simulink model "sh1"  (Simulink 6.6)
settings: Solver=ode45  StartTime=0.0  StopTime=10.0  RelTol=1e-3
libraries: cdsFilt x66, cdsEpicsIn x10, cdsWD x7, cdsMuxMatrix x4, cdsEpicsOut x2, cdsDio x2, dac x1, cdsEpicsBinIn x1, cdsParameters x1
(part 4 of 4)

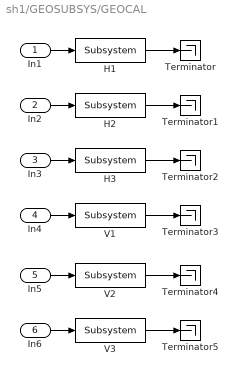
== system sh1/GEOSUBSYS/GEOCAL ==
  In1 : Inport
  In2 : Inport  Port=2
  In3 : Inport  Port=3
  In4 : Inport  Port=4
  In5 : Inport  Port=5
  In6 : Inport  Port=6
  H1 : cdsFilt/Subsystem  Tag=cdsFilt  Description=|  SystemSampleTime=-1
      | Purpose:                                                                                                                                                                                                                                  
      | Standard CDS IIR filter module.                                                                                                                                                                                                           
      |                                                                                                                                                                                                                                           
      | Operation:                                                                                                                                                                                                                                
      | Consists of 10 second order section IIR filters, plus a ramped gain stage. In FE code, also provides pre-defined test points and excitation channel inputs. The filter coefficients are defined in the LIGO system using the 'foton' tool.
      |                                                                                                                                                                                                                                           
      | Usage:                                                                                                                                                                                                                                    
      | Name the part with the desired filter module name.
      settings: AttributesFormatString=%<Tag>
  H2 : cdsFilt/Subsystem  Tag=cdsFilt  Description=|  SystemSampleTime=-1
      | Purpose:                                                                                                                                                                                                                                  
      | Standard CDS IIR filter module.                                                                                                                                                                                                           
      |                                                                                                                                                                                                                                           
      | Operation:                                                                                                                                                                                                                                
      | Consists of 10 second order section IIR filters, plus a ramped gain stage. In FE code, also provides pre-defined test points and excitation channel inputs. The filter coefficients are defined in the LIGO system using the 'foton' tool.
      |                                                                                                                                                                                                                                           
      | Usage:                                                                                                                                                                                                                                    
      | Name the part with the desired filter module name.
      settings: AttributesFormatString=%<Tag>
  H3 : cdsFilt/Subsystem  Tag=cdsFilt  Description=|  SystemSampleTime=-1
      | Purpose:                                                                                                                                                                                                                                  
      | Standard CDS IIR filter module.                                                                                                                                                                                                           
      |                                                                                                                                                                                                                                           
      | Operation:                                                                                                                                                                                                                                
      | Consists of 10 second order section IIR filters, plus a ramped gain stage. In FE code, also provides pre-defined test points and excitation channel inputs. The filter coefficients are defined in the LIGO system using the 'foton' tool.
      |                                                                                                                                                                                                                                           
      | Usage:                                                                                                                                                                                                                                    
      | Name the part with the desired filter module name.
      settings: AttributesFormatString=%<Tag>
  Terminator{,1..5} (6 alike) : Terminator
  V1 : cdsFilt/Subsystem  Tag=cdsFilt  Description=|  SystemSampleTime=-1
      | Purpose:                                                                                                                                                                                                                                  
      | Standard CDS IIR filter module.                                                                                                                                                                                                           
      |                                                                                                                                                                                                                                           
      | Operation:                                                                                                                                                                                                                                
      | Consists of 10 second order section IIR filters, plus a ramped gain stage. In FE code, also provides pre-defined test points and excitation channel inputs. The filter coefficients are defined in the LIGO system using the 'foton' tool.
      |                                                                                                                                                                                                                                           
      | Usage:                                                                                                                                                                                                                                    
      | Name the part with the desired filter module name.
      settings: AttributesFormatString=%<Tag>
  V2 : cdsFilt/Subsystem  Tag=cdsFilt  Description=|  SystemSampleTime=-1
      | Purpose:                                                                                                                                                                                                                                  
      | Standard CDS IIR filter module.                                                                                                                                                                                                           
      |                                                                                                                                                                                                                                           
      | Operation:                                                                                                                                                                                                                                
      | Consists of 10 second order section IIR filters, plus a ramped gain stage. In FE code, also provides pre-defined test points and excitation channel inputs. The filter coefficients are defined in the LIGO system using the 'foton' tool.
      |                                                                                                                                                                                                                                           
      | Usage:                                                                                                                                                                                                                                    
      | Name the part with the desired filter module name.
      settings: AttributesFormatString=%<Tag>
  V3 : cdsFilt/Subsystem  Tag=cdsFilt  Description=|  SystemSampleTime=-1
      | Purpose:                                                                                                                                                                                                                                  
      | Standard CDS IIR filter module.                                                                                                                                                                                                           
      |                                                                                                                                                                                                                                           
      | Operation:                                                                                                                                                                                                                                
      | Consists of 10 second order section IIR filters, plus a ramped gain stage. In FE code, also provides pre-defined test points and excitation channel inputs. The filter coefficients are defined in the LIGO system using the 'foton' tool.
      |                                                                                                                                                                                                                                           
      | Usage:                                                                                                                                                                                                                                    
      | Name the part with the desired filter module name.
      settings: AttributesFormatString=%<Tag>
  wires:
  V2/1 -> Terminator4/1
  V3/1 -> Terminator5/1
  In6/1 -> V3/1
  In5/1 -> V2/1
  H3/1 -> Terminator2/1
  V1/1 -> Terminator3/1
  In4/1 -> V1/1
  In3/1 -> H3/1
  H1/1 -> Terminator/1
  H2/1 -> Terminator1/1
  In2/1 -> H2/1
  In1/1 -> H1/1

== system sh1/WD/1 ==
  In1 : Inport
  In2 : Inport  Port=2
  In3 : Inport  Port=3
  In4 : Inport  Port=4
  In5 : Inport  Port=5
  In6 : Inport  Port=6
  Gain : Gain  Gain=1000
  Ground : Ground
  MAX : cdsEpicsIn/Subsystem  Tag=cdsEpicsIn  Description=|  SystemSampleTime=-1
      | Purpose:                                                                              
      | Create an EPICS input channel connection to the FE realtime controls.                 
      |                                                                                       
      | Operation:                                                                            
      | Outputs value from an EPICS ai record. Value is floating point with a precision of 3..
      |                                                                                       
      | Usage:                                                                                
      | Name the part with the desired EPICS channel name.
      settings: AttributesFormatString=%<Tag>
  Operator{1,3..6} (5 alike) : RelationalOperator  Operator=>  LogicOutDataTypeMode=Boolean
  Operator2 : RelationalOperator  Operator=>  LogicOutDataTypeMode=Boolean  ZeroCross=off
  SWITCH : cdsWD/Subsystem  Description=cdsWD  SystemSampleTime=-1
      settings: AttributesFormatString=%<Description>
  Sum1 : Sum  Inputs=6
  Out1 : Outport
  wires:
  In1/1 -> Operator1/1
  In2/1 -> Operator2/1
  In3/1 -> Operator3/1
  In4/1 -> Operator4/1
  In5/1 -> Operator5/1
  In6/1 -> Operator6/1
  Operator1/1 -> Sum1/1
  Operator2/1 -> Sum1/2
  Operator3/1 -> Sum1/3
  Operator4/1 -> Sum1/4
  Operator5/1 -> Sum1/5
  Operator6/1 -> Sum1/6
  MAX/1 -> Operator1/2, Operator2/2, Operator3/2, Operator4/2, Operator5/2, Operator6/2
  SWITCH/1 -> Out1/1
  Sum1/1 -> Gain/1
  Ground/1 -> SWITCH/2, SWITCH/3, SWITCH/5, SWITCH/4
  Gain/1 -> SWITCH/1

== system sh1/WD/2 ==
  In1 : Inport
  In2 : Inport  Port=2
  In3 : Inport  Port=3
  In4 : Inport  Port=4
  In5 : Inport  Port=5
  In6 : Inport  Port=6
  Gain : Gain  Gain=1000
  Ground : Ground
  MAX : cdsEpicsIn/Subsystem  Tag=cdsEpicsIn  Description=|  SystemSampleTime=-1
      | Purpose:                                                                              
      | Create an EPICS input channel connection to the FE realtime controls.                 
      |                                                                                       
      | Operation:                                                                            
      | Outputs value from an EPICS ai record. Value is floating point with a precision of 3..
      |                                                                                       
      | Usage:                                                                                
      | Name the part with the desired EPICS channel name.
      settings: AttributesFormatString=%<Tag>
  Operator{1..6} (6 alike) : RelationalOperator  Operator=>  LogicOutDataTypeMode=Boolean
  SWITCH : cdsWD/Subsystem  Description=cdsWD  SystemSampleTime=-1
      settings: AttributesFormatString=%<Description>
  Sum1 : Sum  Inputs=6
  Out1 : Outport
  wires:
  In1/1 -> Operator1/1
  In2/1 -> Operator2/1
  In3/1 -> Operator3/1
  In4/1 -> Operator4/1
  In5/1 -> Operator5/1
  In6/1 -> Operator6/1
  Operator1/1 -> Sum1/1
  Operator2/1 -> Sum1/2
  Operator3/1 -> Sum1/3
  Operator4/1 -> Sum1/4
  Operator5/1 -> Sum1/5
  Operator6/1 -> Sum1/6
  MAX/1 -> Operator1/2, Operator2/2, Operator3/2, Operator4/2, Operator5/2, Operator6/2
  SWITCH/1 -> Out1/1
  Ground/1 -> SWITCH/2, SWITCH/3, SWITCH/5, SWITCH/4
  Sum1/1 -> Gain/1
  Gain/1 -> SWITCH/1

== system sh1/WD/3 ==
  In1 : Inport
  In2 : Inport  Port=2
  In3 : Inport  Port=3
  In4 : Inport  Port=4
  In5 : Inport  Port=5
  In6 : Inport  Port=6
  Gain : Gain  Gain=1000
  Ground : Ground
  MAX : cdsEpicsIn/Subsystem  Tag=cdsEpicsIn  Description=|  SystemSampleTime=-1
      | Purpose:                                                                              
      | Create an EPICS input channel connection to the FE realtime controls.                 
      |                                                                                       
      | Operation:                                                                            
      | Outputs value from an EPICS ai record. Value is floating point with a precision of 3..
      |                                                                                       
      | Usage:                                                                                
      | Name the part with the desired EPICS channel name.
      settings: AttributesFormatString=%<Tag>
  Operator{1..6} (6 alike) : RelationalOperator  Operator=>  LogicOutDataTypeMode=Boolean
  SWITCH : cdsWD/Subsystem  Description=cdsWD  SystemSampleTime=-1
      settings: AttributesFormatString=%<Description>
  Sum1 : Sum  Inputs=6
  Out1 : Outport
  wires:
  In1/1 -> Operator1/1
  In2/1 -> Operator2/1
  In3/1 -> Operator3/1
  In4/1 -> Operator4/1
  In5/1 -> Operator5/1
  In6/1 -> Operator6/1
  Operator1/1 -> Sum1/1
  Operator2/1 -> Sum1/2
  Operator3/1 -> Sum1/3
  Operator4/1 -> Sum1/4
  Operator5/1 -> Sum1/5
  Operator6/1 -> Sum1/6
  MAX/1 -> Operator1/2, Operator2/2, Operator3/2, Operator4/2, Operator5/2, Operator6/2
  SWITCH/1 -> Out1/1
  Ground/1 -> SWITCH/2, SWITCH/3, SWITCH/5, SWITCH/4
  Sum1/1 -> Gain/1
  Gain/1 -> SWITCH/1

== system sh1/WD/4 ==
  In1 : Inport
  In2 : Inport  Port=2
  In3 : Inport  Port=3
  Gain : Gain  Gain=1000
  Ground : Ground
  MAX : cdsEpicsIn/Subsystem  Tag=cdsEpicsIn  Description=|  SystemSampleTime=-1
      | Purpose:                                                                              
      | Create an EPICS input channel connection to the FE realtime controls.                 
      |                                                                                       
      | Operation:                                                                            
      | Outputs value from an EPICS ai record. Value is floating point with a precision of 3..
      |                                                                                       
      | Usage:                                                                                
      | Name the part with the desired EPICS channel name.
      settings: AttributesFormatString=%<Tag>
  Operator1 : RelationalOperator  Operator=>  LogicOutDataTypeMode=Boolean
  Operator2 : RelationalOperator  Operator=>  LogicOutDataTypeMode=Boolean
  Operator3 : RelationalOperator  Operator=>  LogicOutDataTypeMode=Boolean  ZeroCross=off
  SWITCH : cdsWD/Subsystem  Description=cdsWD  SystemSampleTime=-1
      settings: AttributesFormatString=%<Description>
  Sum1 : Sum  Inputs=3
  Out1 : Outport
  wires:
  In1/1 -> Operator1/1
  In2/1 -> Operator2/1
  In3/1 -> Operator3/1
  Operator1/1 -> Sum1/1
  Operator2/1 -> Sum1/2
  Operator3/1 -> Sum1/3
  MAX/1 -> Operator1/2, Operator2/2, Operator3/2
  SWITCH/1 -> Out1/1
  Ground/1 -> SWITCH/2, SWITCH/3, SWITCH/5, SWITCH/4
  Sum1/1 -> Gain/1
  Gain/1 -> SWITCH/1

== system sh1/WD/5 ==
  In1 : Inport
  In2 : Inport  Port=2
  Gain : Gain  Gain=1000
  Ground : Ground
  MAX : cdsEpicsIn/Subsystem  Tag=cdsEpicsIn  Description=|  SystemSampleTime=-1
      | Purpose:                                                                              
      | Create an EPICS input channel connection to the FE realtime controls.                 
      |                                                                                       
      | Operation:                                                                            
      | Outputs value from an EPICS ai record. Value is floating point with a precision of 3..
      |                                                                                       
      | Usage:                                                                                
      | Name the part with the desired EPICS channel name.
      settings: AttributesFormatString=%<Tag>
  Operator1 : RelationalOperator  Operator=>  LogicOutDataTypeMode=Boolean
  Operator2 : RelationalOperator  Operator=>  LogicOutDataTypeMode=Boolean
  SWITCH : cdsWD/Subsystem  Description=cdsWD  SystemSampleTime=-1
      settings: AttributesFormatString=%<Description>
  Sum1 : Sum  Inputs=2
  Out1 : Outport
  wires:
  In1/1 -> Operator1/1
  In2/1 -> Operator2/1
  Operator1/1 -> Sum1/1
  Operator2/1 -> Sum1/2
  MAX/1 -> Operator1/2, Operator2/2
  SWITCH/1 -> Out1/1
  Ground/1 -> SWITCH/2, SWITCH/3, SWITCH/5, SWITCH/4
  Sum1/1 -> Gain/1
  Gain/1 -> SWITCH/1

== system sh1/WD/6 ==
  In1 : Inport
  In2 : Inport  Port=2
  In3 : Inport  Port=3
  In4 : Inport  Port=4
  Gain : Gain  Gain=1000
  Ground : Ground
  MAX : cdsEpicsIn/Subsystem  Tag=cdsEpicsIn  Description=|  SystemSampleTime=-1
      | Purpose:                                                                              
      | Create an EPICS input channel connection to the FE realtime controls.                 
      |                                                                                       
      | Operation:                                                                            
      | Outputs value from an EPICS ai record. Value is floating point with a precision of 3..
      |                                                                                       
      | Usage:                                                                                
      | Name the part with the desired EPICS channel name.
      settings: AttributesFormatString=%<Tag>
  Operator{1..4} (4 alike) : RelationalOperator  Operator=>  LogicOutDataTypeMode=Boolean
  SWITCH : cdsWD/Subsystem  Description=cdsWD  SystemSampleTime=-1
      settings: AttributesFormatString=%<Description>
  Sum1 : Sum  Inputs=4
  Out1 : Outport
  wires:
  In1/1 -> Operator1/1
  In2/1 -> Operator2/1
  In3/1 -> Operator3/1
  In4/1 -> Operator4/1
  Operator1/1 -> Sum1/1
  Operator2/1 -> Sum1/2
  Operator3/1 -> Sum1/3
  Operator4/1 -> Sum1/4
  MAX/1 -> Operator1/2, Operator2/2, Operator3/2, Operator4/2
  SWITCH/1 -> Out1/1
  Ground/1 -> SWITCH/2, SWITCH/3, SWITCH/5, SWITCH/4
  Sum1/1 -> Gain/1
  Gain/1 -> SWITCH/1
